simulink model "resourceManagement"  (R2017b)
settings: Solver=FixedStepAuto  StartTime=0.0  StopTime=3600*24  MaxStep=1e-4  RelTol=1e-3
model workspace: external: MATLAB File resourceParam.m (data not in the file)
values from neighbouring files (symbols this model uses):
  c = 1005.4    [resourceParam.m]    (also in resourceParams.mat)
  cost = 2.5E-8    (= 2.5e-08)    [resourceParam.m]    (also in resourceParams.mat)
  costPerKWH = 0.12    [resourceParam.m]
  M = 1778.3691144576505    (= 1778.36911446)    [resourceParam.m]    (also in resourceParams.mat)
  Mdot = 3600    [resourceParam.m]    (also in resourceParams.mat)
  Req = 4.2697563775143509E-7    (= 4.26975637751e-07)    [resourceParam.m]    (also in resourceParams.mat)
  THeater = 50    [resourceParam.m]    (also in resourceParams.mat)
  TinIC = 20    [resourceParam.m]    (also in resourceParams.mat)
libraries: elec_lib x7, nesl_utility x7, fl_lib x6, simulink_extras x3
settings Model: Creator=pjan8  LastModifiedBy=peter

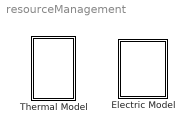
== system resourceManagement ==
  Electric Model : Subsystem
  Thermal Model : Subsystem

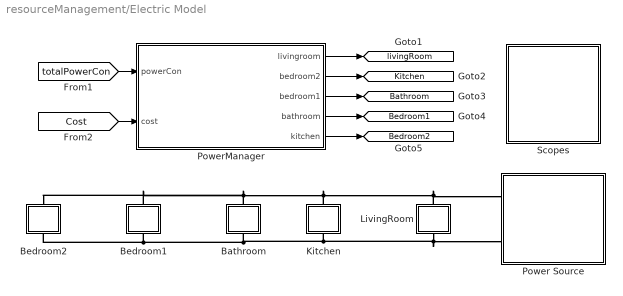
== system resourceManagement/Electric Model ==
  Bathroom : Subsystem
  Bedroom1 : Subsystem
  Bedroom2 : Subsystem
  Kitchen : Subsystem
  LivingRoom : Subsystem
  Power Source : Subsystem
  PowerManager : Stateflow chart  TreatAsAtomicUnit=on
  Scopes : Subsystem
  tag scope: Bathroom=global, Bedroom1=global, Bedroom2=global, Kitchen=global, livingRoom=global
  wires:
  PowerManager/1(livingroom) -> [livingRoom]
  PowerManager/2(bedroom2) -> [Kitchen]
  PowerManager/3(bedroom1) -> [Bathroom]
  PowerManager/4(bathroom) -> [Bedroom1]
  PowerManager/5(kitchen) -> [Bedroom2]
  [totalPowerCon] -> PowerManager/1(powerCon)
  [Cost] -> PowerManager/2(cost)
  connections:
  LivingRoom/LConn1 -- Power Source/LConn1 -- Bedroom1/LConn1 -- Bedroom2/LConn1 -- Bathroom/LConn1 -- Kitchen/LConn1
  LivingRoom/RConn1 -- Bedroom2/RConn1 -- Bedroom1/RConn1 -- Bathroom/RConn1 -- Kitchen/RConn1 -- Power Source/LConn2

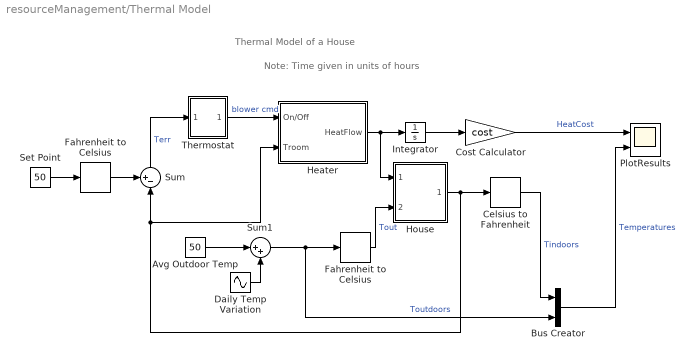
== system resourceManagement/Thermal Model ==
  note: Thermal Model of a House
  note: Note: Time given in units of hours
  Avg Outdoor Temp : Constant  Value=50
  Bus Creator : BusCreator  Inputs=2
  Celsius to Fahrenheit : simulink_extras/Transformations/Celsius to Fahrenheit
      settings: SourceProductName=Simulink  SourceProductBaseCode=SL
  Cost Calculator : Gain  Gain=cost  SaturateOnIntegerOverflow=on  OutDataTypeStr=Inherit: Same as input  ParamDataTypeStr=Inherit: Same as input
  Daily Temp Variation : Sin  Amplitude=15  Frequency=2*pi/24  SampleTime=0
  Fahrenheit to Celsius : simulink_extras/Transformations/Fahrenheit to Celsius
      settings: SourceProductName=Simulink  SourceProductBaseCode=SL
  "Fahrenheit to Celsius " : simulink_extras/Transformations/Fahrenheit to Celsius
      settings: SourceProductName=Simulink  SourceProductBaseCode=SL
  Heater : Subsystem
  House : Subsystem
      mask Display: image(fullfile(matlabroot,'toolbox','simulink','simdemos','simgeneral','images','HouseHeatHousePix.svg'))
  Integrator : Integrator
  PlotResults : Scope  NumInputPorts=2
  Set Point : Constant  Value=50
  Sum : Sum  Inputs=+-|  SaturateOnIntegerOverflow=on  InputSameDT=on  OutDataTypeStr=Inherit: Same as first input
  Sum1 : Sum  Inputs=|++  SaturateOnIntegerOverflow=on  InputSameDT=on  OutDataTypeStr=Inherit: Same as first input
  Thermostat : Subsystem
      mask Display: image(fullfile(matlabroot,'toolbox','simulink','simdemos','simgeneral','images','HouseHeatThermostatPix.svg'))
  wires:
  Celsius to Fahrenheit/1 -> Bus Creator/1  "Tindoors"
  "Fahrenheit to Celsius "/1 -> Sum/1
  House/1(Room Temp Troom) -> Celsius to Fahrenheit/1, Heater/2(Troom), Sum/2
  Cost Calculator/1 -> PlotResults/1  "HeatCost"
  Fahrenheit to Celsius/1 -> House/2(Outdoor Temp Tout)  "Tout"
  Bus Creator/1 -> PlotResults/2  "Temperatures"
  Set Point/1 -> "Fahrenheit to Celsius "/1
  Thermostat/1(Blower switch) -> Heater/1(On/Off)  "blower cmd"
  Daily Temp Variation/1 -> Sum1/2
  Sum1/1 -> Fahrenheit to Celsius/1, Bus Creator/2  "Toutdoors"
  Sum/1 -> Thermostat/1(Terr)  "Terr"
  Avg Outdoor Temp/1 -> Sum1/1
  Integrator/1 -> Cost Calculator/1
  Heater/1(HeatFlow) -> Integrator/1, House/1(Heater QDot In)

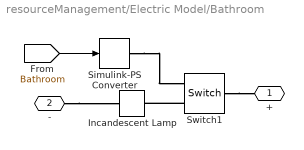
== system resourceManagement/Electric Model/Bathroom ==
  Incandescent Lamp : elec_lib/Passive Devices/Incandescent Lamp  R_param=1  R0=0.15 Ohm  R1=1 Ohm  i0=70 A  i1=10 A  Vrated=12 V  alpha=0.004 1/K  tc=25 ms  initial_state=1  t_fault=inf s  R_fault=1e6 Ohm
      settings: SourceProductName=Simscape Electronics  SourceProductBaseCode=SN
  Simulink-PS Converter : nesl_utility/Simulink-PS Converter  PhysicalDomain=network_engine_domain  SubClassName=ps_input  LeftPortType=input  RightPortType=output  PseudoPeriodic=off  Frequencies=[]  NoiseDistribution=none  NoiseParameters=[]  Unit=1  AffineConversion=off  FilteringAndDerivatives=provide  SimscapeFilterOrder=1  InputFilterTimeConstant=0.001  UdotUserProvided=0
  Switch1 : fl_lib/Electrical/Electrical Elements/Switch  R_closed=0.01 Ohm  G_open=1e-8 1/Ohm  Threshold=0  i_specify=off  i_priority=None  i=0 A  i_nominal_specify=off  i_nominal_unit=A  i_nominal_value=1  v_specify=off  v_priority=None  v=0 V  v_nominal_specify=off  v_nominal_unit=V  v_nominal_value=1
      settings: SourceProductName=Simscape
  + : PMIOPort  Port=1  Side=Left
  - : PMIOPort  Port=2  Side=Right
  wires:
  [Bathroom] -> Simulink-PS Converter/1
  connections:
  Switch1/RConn2 -- Incandescent Lamp/LConn1
  Switch1/LConn1 -- +/RConn1
  -/RConn1 -- Incandescent Lamp/RConn1
  Simulink-PS Converter/RConn1 -- Switch1/RConn1

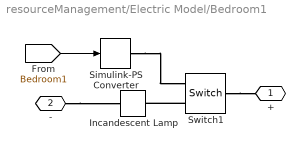
== system resourceManagement/Electric Model/Bedroom1 ==
  Incandescent Lamp : elec_lib/Passive Devices/Incandescent Lamp  R_param=1  R0=0.15 Ohm  R1=1 Ohm  i0=70 A  i1=10 A  Vrated=12 V  alpha=0.004 1/K  tc=25 ms  initial_state=1  t_fault=inf s  R_fault=1e6 Ohm
      settings: SourceProductName=Simscape Electronics  SourceProductBaseCode=SN
  Simulink-PS Converter : nesl_utility/Simulink-PS Converter  PhysicalDomain=network_engine_domain  SubClassName=ps_input  LeftPortType=input  RightPortType=output  PseudoPeriodic=off  Frequencies=[]  NoiseDistribution=none  NoiseParameters=[]  Unit=1  AffineConversion=off  FilteringAndDerivatives=provide  SimscapeFilterOrder=1  InputFilterTimeConstant=0.001  UdotUserProvided=0
  Switch1 : fl_lib/Electrical/Electrical Elements/Switch  R_closed=0.01 Ohm  G_open=1e-8 1/Ohm  Threshold=0  i_specify=off  i_priority=None  i=0 A  i_nominal_specify=off  i_nominal_unit=A  i_nominal_value=1  v_specify=off  v_priority=None  v=0 V  v_nominal_specify=off  v_nominal_unit=V  v_nominal_value=1
      settings: SourceProductName=Simscape
  + : PMIOPort  Port=1  Side=Left
  - : PMIOPort  Port=2  Side=Right
  wires:
  [Bedroom1] -> Simulink-PS Converter/1
  connections:
  Switch1/RConn2 -- Incandescent Lamp/LConn1
  Switch1/LConn1 -- +/RConn1
  -/RConn1 -- Incandescent Lamp/RConn1
  Simulink-PS Converter/RConn1 -- Switch1/RConn1

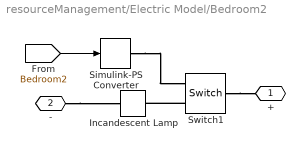
== system resourceManagement/Electric Model/Bedroom2 ==
  Incandescent Lamp : elec_lib/Passive Devices/Incandescent Lamp  R_param=1  R0=0.15 Ohm  R1=1 Ohm  i0=70 A  i1=10 A  Vrated=12 V  alpha=0.004 1/K  tc=25 ms  initial_state=1  t_fault=inf s  R_fault=1e6 Ohm
      settings: SourceProductName=Simscape Electronics  SourceProductBaseCode=SN
  Simulink-PS Converter : nesl_utility/Simulink-PS Converter  PhysicalDomain=network_engine_domain  SubClassName=ps_input  LeftPortType=input  RightPortType=output  PseudoPeriodic=off  Frequencies=[]  NoiseDistribution=none  NoiseParameters=[]  Unit=1  AffineConversion=off  FilteringAndDerivatives=provide  SimscapeFilterOrder=1  InputFilterTimeConstant=0.001  UdotUserProvided=0
  Switch1 : fl_lib/Electrical/Electrical Elements/Switch  R_closed=0.01 Ohm  G_open=1e-8 1/Ohm  Threshold=0  i_specify=off  i_priority=None  i=0 A  i_nominal_specify=off  i_nominal_unit=A  i_nominal_value=1  v_specify=off  v_priority=None  v=0 V  v_nominal_specify=off  v_nominal_unit=V  v_nominal_value=1
      settings: SourceProductName=Simscape
  + : PMIOPort  Port=1  Side=Left
  - : PMIOPort  Port=2  Side=Right
  wires:
  [Bedroom2] -> Simulink-PS Converter/1
  connections:
  Switch1/RConn2 -- Incandescent Lamp/LConn1
  Switch1/LConn1 -- +/RConn1
  -/RConn1 -- Incandescent Lamp/RConn1
  Simulink-PS Converter/RConn1 -- Switch1/RConn1

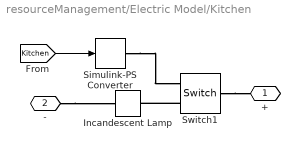
== system resourceManagement/Electric Model/Kitchen ==
  Incandescent Lamp : elec_lib/Passive Devices/Incandescent Lamp  R_param=1  R0=0.15 Ohm  R1=1 Ohm  i0=70 A  i1=10 A  Vrated=12 V  alpha=0.004 1/K  tc=25 ms  initial_state=1  t_fault=inf s  R_fault=1e6 Ohm
      settings: SourceProductName=Simscape Electronics  SourceProductBaseCode=SN
  Simulink-PS Converter : nesl_utility/Simulink-PS Converter  PhysicalDomain=network_engine_domain  SubClassName=ps_input  LeftPortType=input  RightPortType=output  PseudoPeriodic=off  Frequencies=[]  NoiseDistribution=none  NoiseParameters=[]  Unit=1  AffineConversion=off  FilteringAndDerivatives=provide  SimscapeFilterOrder=1  InputFilterTimeConstant=0.001  UdotUserProvided=0
  Switch1 : fl_lib/Electrical/Electrical Elements/Switch  R_closed=0.01 Ohm  G_open=1e-8 1/Ohm  Threshold=0  i_specify=off  i_priority=None  i=0 A  i_nominal_specify=off  i_nominal_unit=A  i_nominal_value=1  v_specify=off  v_priority=None  v=0 V  v_nominal_specify=off  v_nominal_unit=V  v_nominal_value=1
      settings: SourceProductName=Simscape
  + : PMIOPort  Port=1  Side=Left
  - : PMIOPort  Port=2  Side=Right
  wires:
  [Kitchen] -> Simulink-PS Converter/1
  connections:
  Switch1/RConn2 -- Incandescent Lamp/LConn1
  Switch1/LConn1 -- +/RConn1
  -/RConn1 -- Incandescent Lamp/RConn1
  Simulink-PS Converter/RConn1 -- Switch1/RConn1

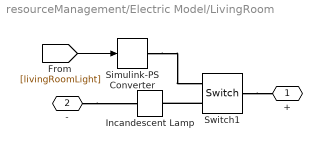
== system resourceManagement/Electric Model/LivingRoom ==
  Incandescent Lamp : elec_lib/Passive Devices/Incandescent Lamp  R_param=1  R0=0.15 Ohm  R1=1 Ohm  i0=70 A  i1=10 A  Vrated=12 V  alpha=0.004 1/K  tc=25 ms  initial_state=1  t_fault=inf s  R_fault=1e6 Ohm
      settings: SourceProductName=Simscape Electronics  SourceProductBaseCode=SN
  Simulink-PS Converter : nesl_utility/Simulink-PS Converter  PhysicalDomain=network_engine_domain  SubClassName=ps_input  LeftPortType=input  RightPortType=output  PseudoPeriodic=off  Frequencies=[]  NoiseDistribution=none  NoiseParameters=[]  Unit=1  AffineConversion=off  FilteringAndDerivatives=provide  SimscapeFilterOrder=1  InputFilterTimeConstant=0.001  UdotUserProvided=0
  Switch1 : fl_lib/Electrical/Electrical Elements/Switch  R_closed=0.01 Ohm  G_open=1e-8 1/Ohm  Threshold=0  i_specify=off  i_priority=None  i=0 A  i_nominal_specify=off  i_nominal_unit=A  i_nominal_value=1  v_specify=off  v_priority=None  v=0 V  v_nominal_specify=off  v_nominal_unit=V  v_nominal_value=1
      settings: SourceProductName=Simscape
  + : PMIOPort  Port=1  Side=Left
  - : PMIOPort  Port=2  Side=Right
  wires:
  [livingRoomLight] -> Simulink-PS Converter/1
  connections:
  Switch1/RConn2 -- Incandescent Lamp/LConn1
  Switch1/LConn1 -- +/RConn1
  -/RConn1 -- Incandescent Lamp/RConn1
  Simulink-PS Converter/RConn1 -- Switch1/RConn1

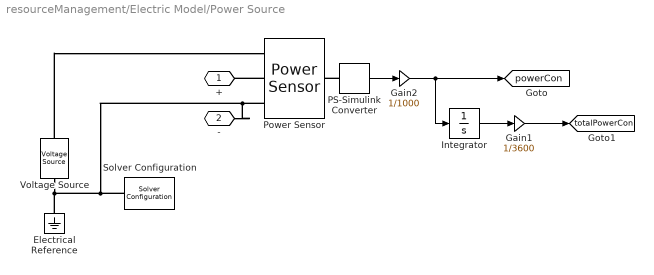
== system resourceManagement/Electric Model/Power Source ==
  Electrical Reference : fl_lib/Electrical/Electrical Elements/Electrical Reference
  Gain1 : Gain  Gain=1/3600
  Gain2 : Gain  Gain=1/1000
  Integrator : Integrator
  PS-Simulink Converter : nesl_utility/PS-Simulink Converter  PhysicalDomain=network_engine_domain  SubClassName=ps_output  LeftPortType=input  RightPortType=output  PseudoPeriodic=off  Frequencies=[]  Unit=1  AffineConversion=off
  Power Sensor : elec_lib/Sensors/Power Sensor  measurement_type=1  averaging_period=1e-4 s
      settings: SourceProductName=Simscape Electronics  SourceProductBaseCode=SN
  Solver Configuration : nesl_utility/Solver Configuration  PhysicalDomain=network_engine_domain  SubClassName=solver  LeftPortType=input  RightPortType=generic  Accelerate=off  Tones=[]  Harmonics=[]  SimulateNoise=off  Profile=off  UseLocalSampling=off  EnableSwitchedLinearOptims=on  FrequencyDomain=off  UseCCode=off  RelTol=0.001  AbsTol=1e-06  MinStep=1e-09  ToWorkspace=off  RevertToSquareIcSolve=off  NumHomotopyIterations=100  PhasorMode=off  PhasorModeNumHarmonics=1  DoDC=off  ResidualTolerance=1e-09  UseLocalSolver=on  LocalSolverChoice=NE_BACKWARD_EULER_ADVANCER  LocalSolverSampleTime=10  DoFixedCost=on  MaxNonlinIter=3  MaxModeIter=2  LinearAlgebra=Sparse  DelaysMemoryBudget=1024  AutomaticFiltering=on  FilteringTimeConstant=0.001
  Voltage Source : elec_lib/Sources/Voltage Source  dc_voltage=12 V  ac_voltage=0 V  ac_shift=0 rad  ac_frequency=60 Hz  noise_mode=0  PSD=0 V^2/Hz  repeatability=1  auto_seed=4177890155  user_seed=0  sample_time=1e-3 s  i_specify=off  i_priority=None  i=0 A  i_nominal_specify=off  i_nominal_unit=A  i_nominal_value=1  v_specify=off  v_priority=None  v=0 V  v_nominal_specify=off  v_nominal_unit=V  v_nominal_value=1
      settings: SourceProductName=Simscape Electronics  SourceProductBaseCode=SN
  + : PMIOPort  Port=1  Side=Left
  - : PMIOPort  Port=2  Side=Left
  tag scope: powerCon=global, totalPowerCon=global
  wires:
  PS-Simulink Converter/1 -> Gain2/1
  Integrator/1 -> Gain1/1
  Gain1/1 -> [totalPowerCon]
  Gain2/1 -> Integrator/1, [powerCon]
  connections:
  Electrical Reference/LConn1 -- Solver Configuration/RConn1 -- -/RConn1 -- Power Sensor/LConn3 -- Voltage Source/RConn1
  PS-Simulink Converter/LConn1 -- Power Sensor/RConn1
  Power Sensor/LConn2 -- +/RConn1
  Voltage Source/LConn1 -- Power Sensor/LConn1

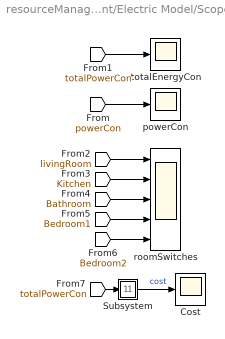
== system resourceManagement/Electric Model/Scopes ==
  Cost : Scope
  Subsystem : Subsystem
  powerCon : Scope
  roomSwitches : Scope  NumInputPorts=5
  totalEnergyCon : Scope
  wires:
  [powerCon] -> powerCon/1
  [livingRoom] -> roomSwitches/1
  [Kitchen] -> roomSwitches/2
  [Bathroom] -> roomSwitches/3
  [Bedroom1] -> roomSwitches/4
  [Bedroom2] -> roomSwitches/5
  [totalPowerCon] -> totalEnergyCon/1
  [totalPowerCon] -> Subsystem/1(In1)
  Subsystem/1(Out1) -> Cost/1  "cost"

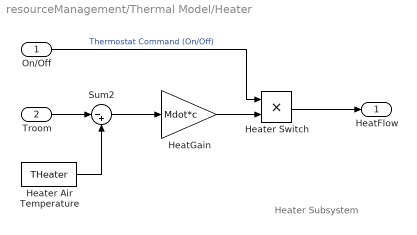
== system resourceManagement/Thermal Model/Heater ==
  note: Heater Subsystem
  On/Off : Inport
  Troom : Inport  Port=2
  HeatGain : Gain  Gain=Mdot*c
  Heater Air Temperature : Constant  Value=THeater
  Heater Switch : Product  RndMeth=Zero
  Sum2 : Sum  Inputs=|-+
  HeatFlow : Outport
  wires:
  Heater Air Temperature/1 -> Sum2/2
  Troom/1 -> Sum2/1
  Sum2/1 -> HeatGain/1
  On/Off/1 -> Heater Switch/1  "Thermostat Command (On/Off)"
  HeatGain/1 -> Heater Switch/2
  Heater Switch/1 -> HeatFlow/1

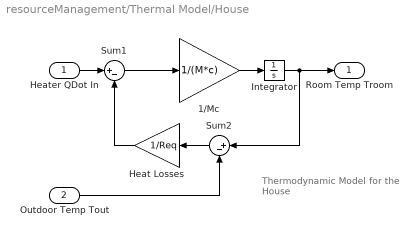
== system resourceManagement/Thermal Model/House ==
  note: Thermodynamic Model
      | for the House
  Heater QDot In : Inport
  Outdoor Temp Tout : Inport  Port=2
  1/Mc : Gain  Gain=1/(M*c)  SaturateOnIntegerOverflow=on  OutDataTypeStr=Inherit: Same as input  ParamDataTypeStr=Inherit: Same as input
  Heat Losses : Gain  Gain=1/Req  SaturateOnIntegerOverflow=on  OutDataTypeStr=Inherit: Same as input  ParamDataTypeStr=Inherit: Same as input
  Integrator : Integrator  InitialCondition=TinIC
  Sum1 : Sum  Inputs=|+-  SaturateOnIntegerOverflow=on  InputSameDT=on  OutDataTypeStr=Inherit: Same as first input
  Sum2 : Sum  Inputs=|+-  SaturateOnIntegerOverflow=on  InputSameDT=on  OutDataTypeStr=Inherit: Same as first input
  Room Temp Troom : Outport  InitialOutput=0
  wires:
  Outdoor Temp Tout/1 -> Sum2/2
  Heater QDot In/1 -> Sum1/1
  Sum1/1 -> 1/Mc/1
  Sum2/1 -> Heat Losses/1
  Heat Losses/1 -> Sum1/2
  1/Mc/1 -> Integrator/1
  Integrator/1 -> Sum2/1, Room Temp Troom/1

== system resourceManagement/Thermal Model/Thermostat ==
  note: Thermostat Subsystem
  Terr : Inport
  Relay1 : Relay  OnSwitchValue=5*(5/9)  OffSwitchValue=-5*(5/9)
  Blower switch : Outport  InitialOutput=0
  wires:
  Terr/1 -> Relay1/1
  Relay1/1 -> Blower switch/1

== system resourceManagement/Electric Model/Scopes/Subsystem ==
  In1 : Inport
  Gain : Gain  Gain=costPerKWH
  Out1 : Outport
  tag scope: Cost=global
  wires:
  Gain/1 -> Out1/1, [Cost]
  In1/1 -> Gain/1

== stateflow chart resourceManagement/Electric Model/PowerManager ==
  state Off
    en:
    livingroom =0;
    kitchen=0;
    bathroom=0;
    bedroom1=0;
    bedroom2=0;
  state idle
  state On
    en:
    livingroom =1;
    kitchen=1;
    bathroom=1;
    bedroom1=1;
    bedroom2=1;
  (junction 28) -> idle
  (default) -> idle
  Off -> (junction 28)
  idle -> Off [order 1] : [cost>costThresh]
  (junction 33) -> (junction 28)
  idle -> On [order 2]
  On -> (junction 33)
  data: powerCon input; livingroom output =1; bedroom2 output =1; bedroom1 output =1; bathroom output =1; kitchen output =1; cost input; costThresh parameter
